simulink model "one_channel_realistic"  (R2022b)
settings: Solver=FixedStepAuto  StartTime=0.0  StopTime=6  FixedStep=1/fs  RelTol=1e-3
values from neighbouring files (symbols this model uses):
  Av_scene = 1    [one_channel_realistic_script.m]
  Num_high = [-8.51268039623e-07 -6.052672635e-07 -8.70010684312e-07 -1.21399654384e-06 -1.65302530712e-06 -2.20472140055e-06 -2.88855427812e-06 -3.7258279046e-06 -4.73963382321e-06 -5.9547629121e-06 -7.39757093819e-06 -9.09579309559e-06 ... (231 elements, 1x231)]    [FIR.mat]    (also in FIR_one_channel_realistic.mat = [0.0171812461017 -0.0043419947643 -0.0037939006674 -0.003290)
  Num_low = [0.00562027911808 0.0373184306138 0.11476696359 0.212679163754 0.259230325849 0.212679163754 0.11476696359 0.0373184306138 0.00562027911808]    [FIR.mat]    (also in FIR_one_channel_realistic.mat = [6.75221820539e-05 8.90946038244e-06 9.44182731134e-06 9.986)
libraries: simulink_extras x1
settings Model: Creator=joaovitor  LastModifiedBy=alunos
settings DataIOCC: ExternalInput=signal

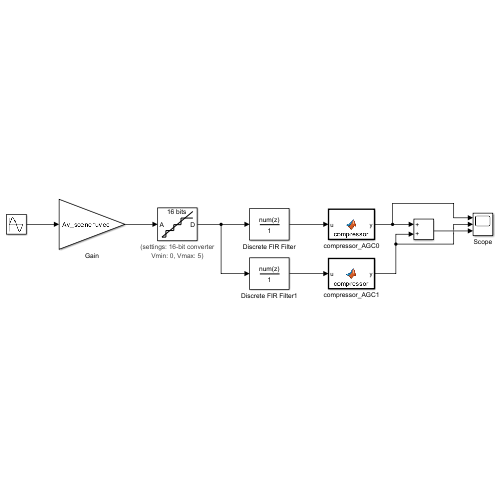
[thumbnail: Simulink's stored preview of the top-level diagram]
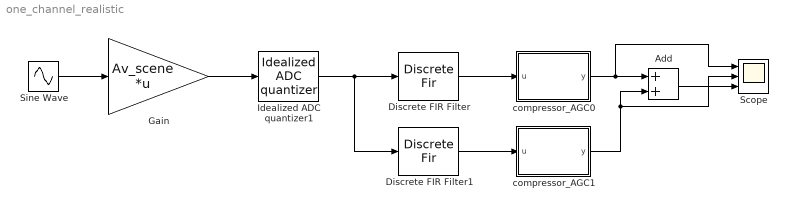
== system one_channel_realistic ==
  Add : Sum
  Discrete FIR Filter : DiscreteFir  Coefficients=Num_low
  Discrete FIR Filter1 : DiscreteFir  Coefficients=Num_high
  Gain : Gain  Gain=Av_scene  Multiplication=Matrix(K*u) (u vector)
  Idealized ADC quantizer1 : simulink_extras/Additional Discrete/Idealized ADC quantizer  NumberOfConverterBits=16  Vmin=0  Vmax=5  OutputDataType=int16  OutputNegativeValues=off
  Scope : Scope  NumInputPorts=3
  Sine Wave : Sin  SampleTime=0
  compressor_AGC0 : MATLAB Function  TreatAsAtomicUnit=on
  compressor_AGC1 : MATLAB Function  TreatAsAtomicUnit=on
  wires:
  Discrete FIR Filter/1 -> compressor_AGC0/1(u)
  Discrete FIR Filter1/1 -> compressor_AGC1/1(u)
  compressor_AGC0/1(y) -> Scope/1, Add/1
  compressor_AGC1/1(y) -> Scope/2, Add/2
  Add/1 -> Scope/3
  Idealized ADC quantizer1/1 -> Discrete FIR Filter1/1, Discrete FIR Filter/1
  Sine Wave/1 -> Gain/1
  Gain/1 -> Idealized ADC quantizer1/1

== matlab function one_channel_realistic/compressor_AGC1 ==
  data: u input; y output
function y = compressor(u)
    % Compressor with Attack and Release
    % u: input signal
    % y: compressed output signal

    % Parameters (adjust these to match your compressor design)
    threshold_dB = -10;  % Threshold in dB
    threshold = 10^(threshold_dB / 20);  % Convert dB to linear scale
    ratio = 2;  % Compression ratio
    attackTime = 0.1;  % Attack time in seconds
    releaseTime = 0.2;  % Release time in seconds
    fs = 10000;  % Sampling frequency (Hz)

    % Initialize persistent variables
    persistent level;
    if isempty(level)
        level = 0;
    end

    % Compute the envelope of the input signal
    abs_u = abs(u);
    if abs_u > level
        % Attack phase
        level = (1 - exp(-1 / (fs * attackTime))) * abs_u + exp(-1 / (fs * attackTime)) * level;
    else
        % Release phase
        level = (1 - exp(-1 / (fs * releaseTime))) * abs_u + exp(-1 / (fs * releaseTime)) * level;
    end

    % Apply compression
    if level > threshold
        gain = threshold + (level - threshold) / ratio;
    else
        gain = level;
    end

    % Apply the computed gain to the input signal
    y = (gain / level) * u;
end

== matlab function one_channel_realistic/compressor_AGC0 ==
  data: u input; y output
function y = compressor(u)
    % Compressor with Attack and Release
    % u: input signal
    % y: compressed output signal

    % Parameters (adjust these to match your compressor design)
    threshold_dB = -10;  % Threshold in dB
    threshold = 10^(threshold_dB / 20);  % Convert dB to linear scale
    ratio = 2;  % Compression ratio
    attackTime = 0.01;  % Attack time in seconds
    releaseTime = 0.02;  % Release time in seconds
    fs = 10000;  % Sampling frequency (Hz)

    % Initialize persistent variables
    persistent level;
    if isempty(level)
        level = 0;
    end

    % Compute the envelope of the input signal
    abs_u = abs(u);
    if abs_u > level
        % Attack phase
        level = (1 - exp(-1 / (fs * attackTime))) * abs_u + exp(-1 / (fs * attackTime)) * level;
    else
        % Release phase
        level = (1 - exp(-1 / (fs * releaseTime))) * abs_u + exp(-1 / (fs * releaseTime)) * level;
    end

    % Apply compression
    if level > threshold
        gain = threshold + (level - threshold) / ratio;
    else
        gain = level;
    end

    % Apply the computed gain to the input signal
    y = (gain / level) * u;
end
